simulink model "BVH2_App_Layer"  (Simulink 5.1)
settings: Solver=ode45  StartTime=0.0  StopTime=10.0  RelTol=1e-3
PreLoadFcn:
  | if exist('tl_preloadfcn','file'), tl_preloadfcn(gcs,95); end
PostLoadFcn:
  | if exist('tl_postloadfcn','file'), tl_postloadfcn(gcs,95); end
InitFcn:
  | if exist('tlds_start','file'), tlds_start(gcs); end
undefined symbols (not defined in the file): built, constant, Constant, DiscreteIntegrator, Gain, in, Logic, Product, Saturate, Sum, Switch
libraries: tllib x71, simulink x1
(part 4 of 4)

== stateflow chart BVH2_Appl_Layer/Subsystem/BVH2_Appl_Layer/Dry_RunningAlarm ==
  state greenState
    entry:
    oDryRun55 = 0 ;
    oDryRun66 = 0;
    Counter = 0;
  state DryRunningAlarm
    state DryRun55
      entry:
      Counter= 0 ;
      oDryRun66 = 0 ;
      oDryRun55 = 1;
      during:
      Counter ++;
    state DryRun66
      entry:
      Counter = 0 ;
      oDryRun66 = 1 ;
      oDryRun55 = 0;
      during:
      Counter++ ;
    DryRun55 -> DryRun66 : [Counter > 400]
    DryRun66 -> DryRun55 : [Counter > 400]
  greenState -> DryRun66 : [iDryRunAlarm == 1  ]
  (default) -> greenState : [iDryRunAlarm == 0]
  DryRunningAlarm -> greenState : [iDryRunAlarm == 0]
  data: iDryRunAlarm input boolean; oDryRun55 output boolean; oDryRun66 output boolean; Counter local uint16
